simulink model "DCpanel"  (Simulink 9.0)
settings: Solver=ode45  StartTime=0.0  StopTime=10.0  MaxStep=1e-3  RelTol=1e-6  EnableMultiTasking=on
values from neighbouring files (symbols this model uses):
  B = 1    [DCmach_DirectStartSim_CompMeas_Lab.m]    (also in DCmach_DirectStartSim_PreLab.m = 0.004)
  J = 1    [DCmach_DirectStartSim_CompMeas_Lab.m]    (also in DCmach_DirectStartSim_PreLab.m = 0.05)
  La = 1    [DCmach_DirectStartSim_CompMeas_Lab.m]    (also in DCmach_DirectStartSim_PreLab.m = 19.85)
  lambda = K_lambda*ifeild    (= 1.5)    [DCmach_DirectStartSim_CompMeas_Lab.m]    (also in DCmach_DirectStartSim_PreLab.m = 1.1394)
  Ra = 1    [DCmach_DirectStartSim_CompMeas_Lab.m]    (also in DCmach_DirectStartSim_PreLab.m = 1.9)
  TL_step = 0    [DCmach_DirectStartSim_PreLab.m]
  TL_steptime1 = 0    [DCmach_DirectStartSim_PreLab.m]
  TL_steptime2 = 0    [DCmach_DirectStartSim_PreLab.m]
  vT_step = mean(vT_mes(num2))    [DCmach_DirectStartSim_CompMeas_Lab.m]    (also in DCmach_DirectStartSim_PreLab.m = 180)
  vT_steptime = time_mes(num1(1))    [DCmach_DirectStartSim_CompMeas_Lab.m]    (also in DCmach_DirectStartSim_PreLab.m = 0.1)
settings Model: Creator=andlinds  LastModifiedBy=emmag
settings DataIOCC: LimitDataPoints=on  SignalLoggingSaveFormat=ModelDataLogs
settings OptimizationCC: ExpressionDepthLimit=2147483647  InitFltsAndDblsToZero=on
settings DebuggingCC: FcnCallInpInsideContextMsg=warning  StateNameClashWarn=warning  StrictBusMsg=Warning
settings GRTTargetCC: GeneratePreprocessorConditionals=Disable all  CombineOutputUpdateFcns=off  GRTInterface=on

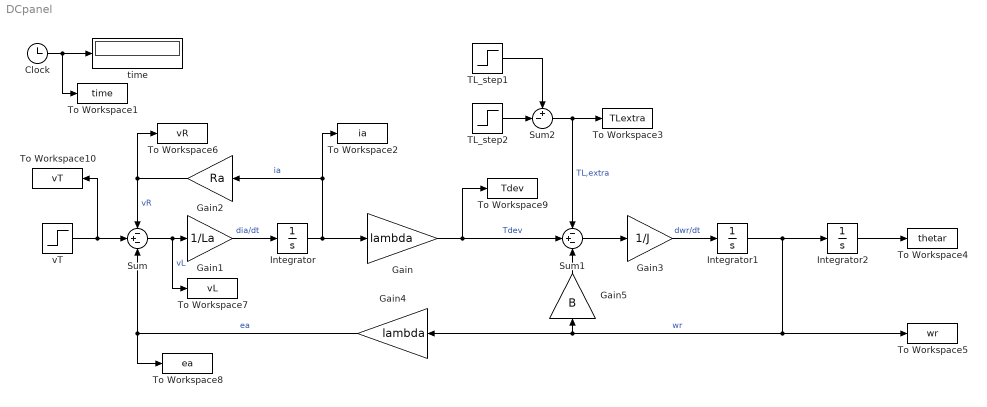
== system DCpanel ==
  Clock : Clock
  Gain : Gain  Gain=lambda
  Gain1 : Gain  Gain=1/La
  Gain2 : Gain  Gain=Ra
  Gain3 : Gain  Gain=1/J
  Gain4 : Gain  Gain=lambda
  Gain5 : Gain  Gain=B
  Integrator : Integrator
  Integrator1 : Integrator
  Integrator2 : Integrator
  Sum : Sum  Inputs=-+-
  Sum1 : Sum  Inputs=-+-
  Sum2 : Sum  Inputs=+-|
  TL_step1 : Step  Time=TL_steptime1  After=TL_step  SampleTime=0
  TL_step2 : Step  Time=TL_steptime2  After=TL_step*2  SampleTime=0
  To Workspace1 : ToWorkspace  VariableName=time  SampleTime=-1
  To Workspace10 : ToWorkspace  VariableName=vT  SampleTime=-1
  To Workspace2 : ToWorkspace  VariableName=ia  SampleTime=-1
  To Workspace3 : ToWorkspace  VariableName=TLextra  SampleTime=-1
  To Workspace4 : ToWorkspace  VariableName=thetar  SampleTime=-1
  To Workspace5 : ToWorkspace  VariableName=wr  SampleTime=-1
  To Workspace6 : ToWorkspace  VariableName=vR  SampleTime=-1
  To Workspace7 : ToWorkspace  VariableName=vL  SampleTime=-1
  To Workspace8 : ToWorkspace  VariableName=ea  SampleTime=-1
  To Workspace9 : ToWorkspace  VariableName=Tdev  SampleTime=-1
  time : Display
  vT : Step  Time=vT_steptime  After=vT_step  SampleTime=0
  wires:
  Clock/1 -> time/1, To Workspace1/1
  Integrator/1 -> Gain/1, Gain2/1, To Workspace2/1  "ia"
  Gain/1 -> Sum1/2, To Workspace9/1  "Tdev"
  vT/1 -> Sum/2, To Workspace10/1
  Gain1/1 -> Integrator/1  "dia/dt"
  Sum/1 -> Gain1/1, To Workspace7/1  "vL"
  Gain2/1 -> Sum/1, To Workspace6/1  "vR"
  TL_step2/1 -> Sum2/2
  TL_step1/1 -> Sum2/1
  Sum2/1 -> Sum1/1, To Workspace3/1  "TL,extra"
  Gain3/1 -> Integrator1/1  "dwr/dt"
  Sum1/1 -> Gain3/1
  Integrator1/1 -> Integrator2/1, To Workspace5/1, Gain4/1, Gain5/1  "wr"
  Integrator2/1 -> To Workspace4/1
  Gain4/1 -> Sum/3, To Workspace8/1  "ea"
  Gain5/1 -> Sum1/3
